simulink model "Script_es2_1"  (R2023b)
settings: Solver=VariableStepAuto  StartTime=0.0  StopTime=30  RelTol=1e-3
libraries: dspfdesign x8, vrlib x2
settings Model: Creator=bolla  LastModifiedBy=bolla

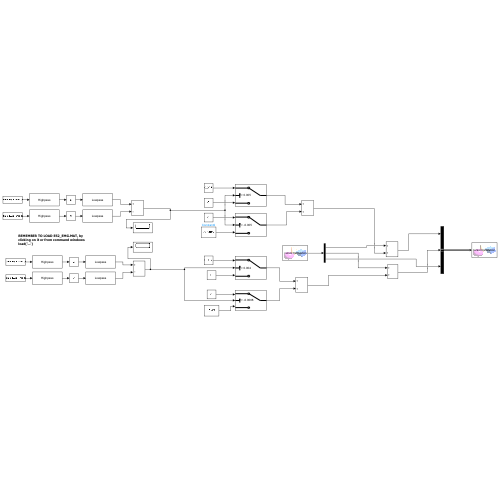
[thumbnail: Simulink's stored preview of the top-level diagram]
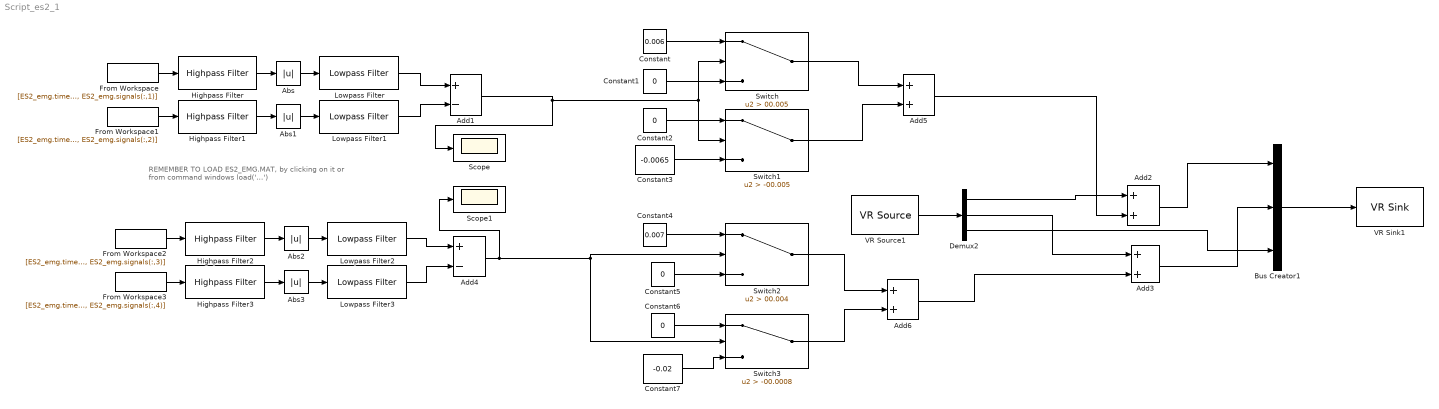
== system Script_es2_1 ==
  note: REMEMBER TO LOAD ES2_EMG.MAT, by clicking on it or from command windows load('...')
  Abs{,1..3} (4 alike) : Abs  SaturateOnIntegerOverflow=off
  Add1 : Sum  Inputs=+-
  Add{2..3,5..6} (4 alike) : Sum
  Add4 : Sum  Inputs=+-
  Bus Creator1 : BusCreator  Inputs=3
  Constant : Constant  Value=0.006
  Constant{1..2,5..6} (4 alike) : Constant  Value=0
  Constant3 : Constant  Value=-0.0065
  Constant4 : Constant  Value=0.007
  Constant7 : Constant  Value=-0.02
  Demux2 : Demux  Outputs=3
  From Workspace : FromWorkspace  VariableName=[ES2_emg.time, ES2_emg.signals(:,1)]  SampleTime=0.001
  From Workspace1 : FromWorkspace  VariableName=[ES2_emg.time, ES2_emg.signals(:,2)]  SampleTime=0.001
  From Workspace2 : FromWorkspace  VariableName=[ES2_emg.time, ES2_emg.signals(:,3)]  SampleTime=0.001
  From Workspace3 : FromWorkspace  VariableName=[ES2_emg.time, ES2_emg.signals(:,4)]  SampleTime=0.001
  Highpass Filter{,1..3} (4 alike) : dspfdesign/Highpass Filter  FilterType=FIR  DesignForMinimumOrder=on  FilterOrder=50  StopbandFrequency=30  PassbandFrequency=450  StopbandAttenuation=80  PassbandRipple=0.1  SampleRate=44100  SimulateUsing=Interpreted execution  roundingMode=Floor  coeffsDataTypeStr=fixdt(1,16)
  Lowpass Filter{,1..3} (4 alike) : dspfdesign/Lowpass Filter  FilterType=FIR  DesignForMinimumOrder=on  FilterOrder=50  PassbandFrequency=3  StopbandFrequency=6  PassbandRipple=0.1  StopbandAttenuation=80  SampleRate=44100  SimulateUsing=Interpreted execution  roundingMode=Floor  coeffsDataTypeStr=fixdt(1,16)
  Scope : Scope
  Scope1 : Scope
  Switch : Switch  Criteria=u2 > Threshold  Threshold=00.005  SaturateOnIntegerOverflow=off  InputSameDT=off
  Switch1 : Switch  Criteria=u2 > Threshold  Threshold=-00.005  SaturateOnIntegerOverflow=off  InputSameDT=off
  Switch2 : Switch  Criteria=u2 > Threshold  Threshold=00.004  SaturateOnIntegerOverflow=off  InputSameDT=off
  Switch3 : Switch  Criteria=u2 > Threshold  Threshold=-00.0008  SaturateOnIntegerOverflow=off  InputSameDT=off
  VR Sink1 : vrlib/VR Sink  InstantiateOnLoad=on  SampleTime=0.1  ViewEnable=on  RemoteChange=off  RemoteView=off  FieldsWritten=cursor.translation.3.1.1.double  WorldFileName=8_palline_color.wrl  AutoView=off  VideoDimensions=[]  AllowVariableSize=off
  VR Source1 : vrlib/VR Source  InstantiateOnLoad=on  SampleTime=0.1  ViewEnable=on  RemoteChange=off  RemoteView=off  FieldsRead=cursor.translation.1.3.1.double  WorldFileName=8_palline_color.wrl  AutoView=off  VideoDimensions=[]  AllowVariableSize=off  FigureProperties="{'Position', 'Name', 'Viewpoint', 'CameraBound', 'CameraDirection', 'CameraPosition', 'CameraUpVector', 'ZoomFactor', 'Antialiasing', 'Headlight', 'Lighting', 'NavPanel', 'Sound', 'StatusBar', 'Stereo3D', 'Stereo3DCameraOffset', 'Stereo3DHIT', 'ToolBar', 'Textures', 'Transparency', 'Triad', 'Wireframe', 'NavZones', 'NavMode', 'NavSpeed', 'CaptureFileFormat', 'CaptureFileName', 'Record2DCompressMethod', 'Record2DCompressQuality', 'Record2D', 'Record2DFileName', 'Record2DFPS'; [6.4900000000000000e+02   3.2400000000000000e+02   5.7600000000000000e+02   3.5000000000000000e+02], '', '_untitled_1', 'on', [0.0000000000000000e+00   0.0000000000000000e+00  -1.0000000000000000e+00], [0.0000000000000000e+00   0.0000000000000000e+00   0.0000000000000000e+00], [0.0000000000000000e+00   1.0000000000000000e+00   0.0000000000000000e+00], [1.0000000000000000e+00], 'on', 'on', 'on', 'halfbar', 'on', 'on', 'off', [1.0000000149011612e-01], [0.0000000000000000e+00], 'on', 'on', 'on', 'none', 'off', 'off', 'fly', 'normal', 'tif', '%f_anim_%n.tif', 'auto', [7.5000000000000000e+01], 'off', '%f_anim_%n.avi', 'auto'}"
  wires:
  Demux2/3 -> Bus Creator1/3
  Add3/1 -> Bus Creator1/2
  Demux2/1 -> Add2/1
  Add2/1 -> Bus Creator1/1
  Demux2/2 -> Add3/1
  VR Source1/1 -> Demux2/1
  Bus Creator1/1 -> VR Sink1/1
  From Workspace/1 -> Highpass Filter/1
  Highpass Filter/1 -> Abs/1
  Abs/1 -> Lowpass Filter/1
  Highpass Filter1/1 -> Abs1/1
  Abs1/1 -> Lowpass Filter1/1
  From Workspace1/1 -> Highpass Filter1/1
  From Workspace3/1 -> Highpass Filter3/1
  Abs3/1 -> Lowpass Filter3/1
  Highpass Filter3/1 -> Abs3/1
  Highpass Filter2/1 -> Abs2/1
  Abs2/1 -> Lowpass Filter2/1
  From Workspace2/1 -> Highpass Filter2/1
  Lowpass Filter/1 -> Add1/1
  Lowpass Filter1/1 -> Add1/2
  Add1/1 -> Switch1/2, Switch/2, Scope/1
  Lowpass Filter2/1 -> Add4/1
  Lowpass Filter3/1 -> Add4/2
  Constant/1 -> Switch/1
  Constant1/1 -> Switch/3
  Constant2/1 -> Switch1/1
  Constant3/1 -> Switch1/3
  Switch/1 -> Add5/1
  Switch1/1 -> Add5/2
  Add5/1 -> Add2/2
  Switch2/1 -> Add6/1
  Constant7/1 -> Switch3/3
  Constant6/1 -> Switch3/1
  Switch3/1 -> Add6/2
  Add4/1 -> Switch3/2, Switch2/2, Scope1/1
  Constant4/1 -> Switch2/1
  Constant5/1 -> Switch2/3
  Add6/1 -> Add3/2
